simulink model "Caishidianlu_analysis_tu"  (R2020b)
settings: Solver=VariableStepAuto  StartTime=0.0  StopTime=10  RelTol=1e-3
settings Model: Creator=19017  LastModifiedBy=19017
settings OptimizationCC: LifeSpan=inf
settings DebuggingCC: ArithmeticOperatorsInVariantConditions=warning
settings SFSimCC: CustomCodeUndefinedFunction=UseInterfaceOnly
settings CodeAppCC: StateflowObjectComments=on

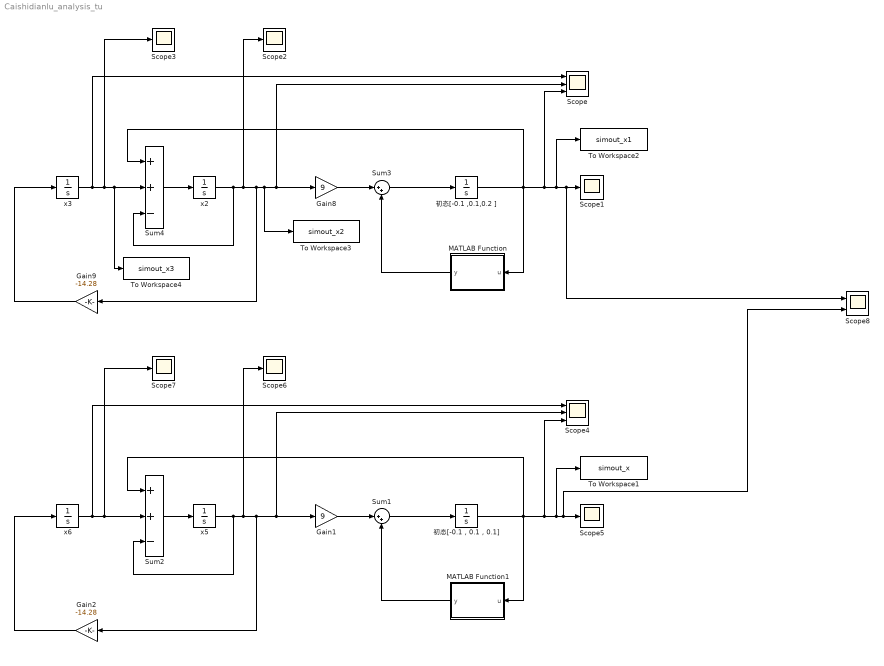
== system Caishidianlu_analysis_tu ==
  Gain1 : Gain  Gain=9
  Gain2 : Gain  Gain=-14.28
  Gain8 : Gain  Gain=9
  Gain9 : Gain  Gain=-14.28
  MATLAB Function : MATLAB Function  TreatAsAtomicUnit=on
  MATLAB Function1 : MATLAB Function  TreatAsAtomicUnit=on
  Scope : Scope  NumInputPorts=3
  Scope{1..3,5..7} (6 alike) : Scope
  Scope4 : Scope  NumInputPorts=3
  Scope8 : Scope  NumInputPorts=2
  Sum1 : Sum  Inputs=|++
  Sum2 : Sum  Inputs=++-
  Sum3 : Sum  Inputs=|++
  Sum4 : Sum  Inputs=++-
  To Workspace1 : ToWorkspace  VariableName=simout_x  SaveFormat=Timeseries  SampleTime=-1
  To Workspace2 : ToWorkspace  VariableName=simout_x1  SampleTime=-1
  To Workspace3 : ToWorkspace  VariableName=simout_x2  SampleTime=-1
  To Workspace4 : ToWorkspace  VariableName=simout_x3  SampleTime=-1
  x2 : Integrator  InitialCondition=0.1
  x3 : Integrator  InitialCondition=0.2
  x5 : Integrator  InitialCondition=0.1
  x6 : Integrator  InitialCondition=0.1
  初态[-0.1 ,0.1,0.2 ] : Integrator  InitialCondition=-0.1
  初态[-0.1，0.1，0.1] : Integrator  InitialCondition=-0.1
  wires:
  x3/1 -> Scope/1, Scope3/1, To Workspace4/1, Sum4/2
  MATLAB Function/1(y) -> Sum3/2
  Gain9/1 -> x3/1
  Gain8/1 -> Sum3/1
  Sum4/1 -> x2/1
  初态[-0.1 ,0.1,0.2 ]/1 -> MATLAB Function/1(u), Scope/3, To Workspace2/1, Scope8/1, Scope1/1, Sum4/1
  Sum3/1 -> 初态[-0.1 ,0.1,0.2 ]/1
  x2/1 -> Sum4/3, Scope2/1, Gain9/1, To Workspace3/1, Scope/2, Gain8/1
  x5/1 -> Sum2/3, Scope6/1, Gain2/1, Scope4/2, Gain1/1
  Sum1/1 -> 初态[-0.1，0.1，0.1]/1
  Sum2/1 -> x5/1
  Gain1/1 -> Sum1/1
  Gain2/1 -> x6/1
  初态[-0.1，0.1，0.1]/1 -> MATLAB Function1/1(u), Scope4/3, To Workspace1/1, Scope8/2, Scope5/1, Sum2/1
  MATLAB Function1/1(y) -> Sum1/2
  x6/1 -> Scope4/1, Scope7/1, Sum2/2

== matlab function Caishidianlu_analysis_tu/MATLAB Function ==
  data: u input; y output
function y = fcn(u)
x1=u;
x1dao=-((2*9)/7)*x1+(((9*3)/7)/2)*(abs(x1+1)-abs(x1-1))
y=x1dao;

== matlab function Caishidianlu_analysis_tu/MATLAB Function1 ==
  data: u input; y output
function y = fcn(u)
x1=u;
x1dao=-((2*9)/7)*x1+(((9*3)/7)/2)*(abs(x1+1)-abs(x1-1))
y=x1dao;
